simulink model "ADRCFirstOrder"  (R2019b)
settings: Solver=VariableStepAuto  StartTime=0.0  StopTime=10  FixedStep=1  MaxStep=0.16  RelTol=1e-3
undefined symbols (not defined in the file): A, Aaobs, B, b0, Baobs, C, Caobs, D, Daobs, Kp
libraries: simulink x1
settings Model: Creator=didi  LastModifiedBy=didi
settings DebuggingCC: ReadBeforeWriteMsg=DisableAll  WriteAfterWriteMsg=DisableAll  WriteAfterReadMsg=DisableAll  MultiTaskDSMMsg=none
settings ModelReferenceCC: UpdateModelReferenceTargets=IfOutOfDate
settings SFSimCC: SFSimEcho=off

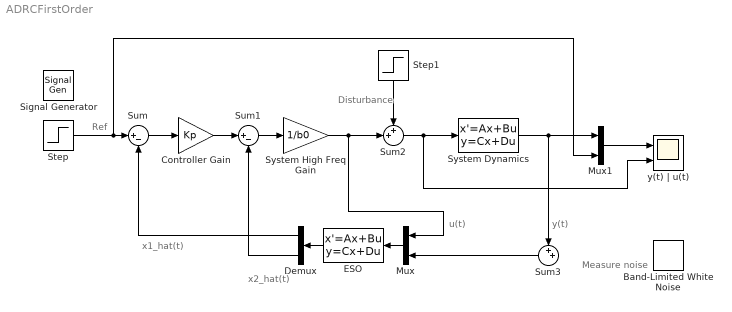
== system ADRCFirstOrder ==
  note: Disturbance
  note: x2_hat(t)
  note: u(t)
  note: Ref
  note: x1_hat(t)
  note: Measure noise
  note: y(t)
  Band-Limited White Noise : simulink/Sources/Band-Limited White Noise  Cov=[0.000001]  Ts=0.76  seed=[23341]
  Controller Gain : Gain  Gain=Kp
  Demux : Demux  Outputs=2
  ESO : StateSpace  A=Aaobs  B=Baobs  C=Caobs  D=Daobs  InitialCondition=0
  Mux : Mux  Inputs=2
  Mux1 : Mux  Inputs=2
  Signal Generator : SignalGenerator  Frequency=0.5
  Step : Step  SampleTime=0
  Step1 : Step  Time=5  After=5  SampleTime=0
  Sum : Sum  Inputs=|+-
  Sum1 : Sum  Inputs=|+-
  Sum2 : Sum  Inputs=++|
  Sum3 : Sum  Inputs=++|
  System Dynamics : StateSpace  A=A  B=B  C=C  D=D  InitialCondition=0
  System High Freq Gain : Gain  Gain=1/b0
  y(t) | u(t) : Scope  NumInputPorts=2
  wires:
  Mux/1 -> ESO/1
  Sum/1 -> Controller Gain/1
  ESO/1 -> Demux/1
  Controller Gain/1 -> Sum1/1
  Demux/2 -> Sum1/2
  Sum1/1 -> System High Freq Gain/1
  System Dynamics/1 -> Sum3/1, Mux1/1
  System High Freq Gain/1 -> Mux/1, Sum2/2
  Sum2/1 -> y(t) | u(t)/2, System Dynamics/1
  Mux1/1 -> y(t) | u(t)/1
  Demux/1 -> Sum/2
  Sum3/1 -> Mux/2
  Step1/1 -> Sum2/1
  Step/1 -> Mux1/2, Sum/1
